simulink model "MIL4L3_SW6_V1_20220211"  (R2018b)
settings: Solver=FixedStepAuto  StartTime=0.0  StopTime=inf  FixedStep=0.001  RelTol=1e-3
PreLoadFcn:
  | A0_MILtest;
undefined symbols (not defined in the file or in its folder): Clb_ICADirect_LaneDisp_StateFive, Clb_ICADirect_LaneDisp_StateFour, Clb_ICADirect_LaneDisp_StateOne, Clb_ICADirect_LaneDisp_StateThree, Clb_ICADirect_LaneDisp_StateTwo, Clb_ICADirect_LaneDisp_StateZero, Clb_ICADirect_LaneDispSW, Clb_ICADirect_TrnLghtsCom_Switch, Clb_ICADirect_TrnLghtsCom_Value, Clb_ICADirect_TrnLghtsCrtl_Inhb, IMAP_Clb_ACU_Driver_Belt, IMAP_Clb_ACU_Driver_Belt_Over, IMAP_Clb_ACU_Passenger_Belt, IMAP_Clb_ACU_Passenger_Belt_Over, IMAP_Clb_ACU_RearLeft_Belt, IMAP_Clb_ACU_RearLeft_Belt_Over, IMAP_Clb_ACU_RearMiddle_Belt, IMAP_Clb_ACU_RearMiddle_Belt_Over, IMAP_Clb_ACU_RearRight_Belt, IMAP_Clb_ACU_RearRight_Belt_Over, IMAP_Clb_AEB_Switch, IMAP_Clb_AEB_Switch_Over, IMAP_Clb_ALC_TLC_Mode, IMAP_Clb_ALC_TLC_Mode_Over, IMAP_Clb_BCM_Battery_Voltage, IMAP_Clb_BCM_Battery_Voltage_Over, IMAP_Clb_BCM_BrakeLamp_State, IMAP_Clb_BCM_BrakeLamp_State_Over, IMAP_Clb_BCM_CHMSL_Status, IMAP_Clb_BCM_CHMSL_Status_Over, IMAP_Clb_BCM_Door_Lock_State, IMAP_Clb_BCM_Door_Lock_State_Over, IMAP_Clb_BCM_FrontWiper_State, IMAP_Clb_BCM_FrontWiper_State_Over, IMAP_Clb_BCM_FrontWiper_Switch, IMAP_Clb_BCM_FrontWiper_Switch_Over, IMAP_Clb_BCM_HazardLamp, IMAP_Clb_BCM_HazardLamp_Over, IMAP_Clb_BCM_HazardLamp_Switch, IMAP_Clb_BCM_HazardLamp_Switch_Over, IMAP_Clb_BCM_HighBeam_State, IMAP_Clb_BCM_HighBeam_State_Over, IMAP_Clb_BCM_Ignition_State, IMAP_Clb_BCM_Ignition_State_Over, IMAP_Clb_BCM_IHBC_Enabled, IMAP_Clb_BCM_IHBC_Enabled_Over, IMAP_Clb_BCM_Left_Light, IMAP_Clb_BCM_Left_Light_Over, IMAP_Clb_BCM_LeftTurn_Switch, IMAP_Clb_BCM_LeftTurn_Switch_Over, IMAP_Clb_BCM_LF_Door_State, IMAP_Clb_BCM_LF_Door_State_Over, IMAP_Clb_BCM_LowBeam_State, IMAP_Clb_BCM_LowBeam_State_Over, IMAP_Clb_BCM_LR_Door_State, IMAP_Clb_BCM_LR_Door_State_Over, IMAP_Clb_BCM_RF_Door_State, IMAP_Clb_BCM_RF_Door_State_Over, IMAP_Clb_BCM_Right_Light, IMAP_Clb_BCM_Right_Light_Over ... (+547)
libraries: CarMaker4SL x2153, simulink x292, dspstat3 x3, canmsglib x2, simulink_extras x1
(part 5 of 52)

== system MIL4L3_SW6_V1_20220211/CarMaker/VehicleControl/SwitchForRealECU_Steering_Angle ==
  In1 : Inport
  Inport : Inport  Port=2
  Compare To Constant1 : simulink/Logic and Bit Operations/Compare To Constant  relop===  const=2  OutDataTypeStr=boolean
  Compare To Constant2 : simulink/Logic and Bit Operations/Compare To Constant  relop===  const=4  OutDataTypeStr=boolean
  Define CM Dict3 : CarMaker4SL/Define CM Dict  xname=User.IO.In.SteeringAngle_Gain  xmono=off  xtype=Double4  xdvaplace=IO_In  xnstates=0  xfirststate=0  xinitial=1
  Define CM Dict4 : CarMaker4SL/Define CM Dict  xname=User.IO.In.SteeringAngle_SW  xmono=off  xtype=Double4  xdvaplace=IO_In  xnstates=0  xfirststate=0  xinitial=0
  Define CM Dict5 : CarMaker4SL/Define CM Dict  xname=User.IO.In.SteeringAngle_SW_Value  xmono=off  xtype=Double4  xdvaplace=IO_In  xnstates=0  xfirststate=0  xinitial=0
  Gain1 : Gain  Gain=pi/180
  Logical Operator : Logic  Operator=OR  AllPortsSameDT=off  OutDataTypeStr=boolean
  Product1 : Product
  Read CM Dict1 : CarMaker4SL/Read CM Dict  xname=User.IO.In.SteeringAngle_SW  xsync=off
  Read CM Dict2 : CarMaker4SL/Read CM Dict  xname=User.IO.In.SteeringAngle_Gain  xsync=off
  Read CM Dict3 : CarMaker4SL/Read CM Dict  xname=User.IO.In.SteeringAngle_SW_Value  xsync=off
  Read CM Dict4 : CarMaker4SL/Read CM Dict  xname=User.IO.In.ADAS_ICAStatusIcon  xsync=off
  Read CM Dict6 : CarMaker4SL/Read CM Dict  xname=User.IO.In.ADAS_LKAState  xsync=off
  Subsystem1 : Subsystem
  Switch1 : Switch  Criteria=u2 > Threshold  Threshold=0.5
  Switch2 : Switch  Criteria=u2 > Threshold  Threshold=0.5
  Out1 : Outport
  wires:
  In1/1 -> Switch1/3
  Read CM Dict4/1 -> Compare To Constant1/1
  Inport/1 -> Gain1/1
  Read CM Dict2/1 -> Product1/2
  Product1/1 -> Switch1/1
  Switch2/1 -> Out1/1
  Switch1/1 -> Switch2/3
  Read CM Dict1/1 -> Switch2/2
  Read CM Dict3/1 -> Switch2/1
  Gain1/1 -> Product1/1, Subsystem1/1(In1)
  Read CM Dict6/1 -> Compare To Constant2/1
  Compare To Constant1/1 -> Logical Operator/1
  Logical Operator/1 -> Switch1/2
  Compare To Constant2/1 -> Logical Operator/2

== system MIL4L3_SW6_V1_20220211/CarMaker/VehicleControl/SwitchForRealECU_Steering_Angle1 ==
  Torque : Inport
  User.IO.In.ADAS_ESATorqueReq : Inport  Port=2
  Compare To Constant1 : simulink/Logic and Bit Operations/Compare To Constant  relop===  const=4  OutDataTypeStr=boolean
  Read CM Dict4 : CarMaker4SL/Read CM Dict  xname=User.IO.In.ADAS_ESAState  xsync=off
  Switch1 : Switch  Criteria=u2 > Threshold  Threshold=0.5
  Out1 : Outport
  wires:
  User.IO.In.ADAS_ESATorqueReq/1 -> Switch1/1
  Compare To Constant1/1 -> Switch1/2
  Read CM Dict4/1 -> Compare To Constant1/1
  Switch1/1 -> Out1/1
  Torque/1 -> Switch1/3

== system MIL4L3_SW6_V1_20220211/CarMaker/VehicleControl/Traffic Attribution Define1 ==
  T00 : Subsystem
  T01 : Subsystem
  T02 : Subsystem
  T03 : Subsystem
  T04 : Subsystem
  T05 : Subsystem
  T06 : Subsystem
  T07 : Subsystem
  T08 : Subsystem
  T09 : Subsystem
  T10 : Subsystem
  T11 : Subsystem
  T12 : Subsystem
  T13 : Subsystem
  T14 : Subsystem
  T15 : Subsystem
  T16 : Subsystem
  T17 : Subsystem
  T18 : Subsystem
  T19 : Subsystem
  T20 : Subsystem
  T21 : Subsystem
  T22 : Subsystem
  T23 : Subsystem

== system MIL4L3_SW6_V1_20220211/CarMaker/VehicleControl/User.IO.In ==
  note: LKA
  note: JA
  note: FDMM
  note: AEB
  note: ESA
  note: EWWW
  note: ELK
  note: ACC
  Define CM Dict : CarMaker4SL/Define CM Dict  xname=User.IO.In.ACCSve_d_ACC_State  xmono=off  xtype=UInt  xdvaplace=None  xnstates=0  xfirststate=0  xinitial=0
  Define CM Dict1 : CarMaker4SL/Define CM Dict  xname=User.IO.In.ACCSve_g_ACC_DecReq  xmono=off  xtype=UInt  xdvaplace=None  xnstates=0  xfirststate=0  xinitial=0
  Define CM Dict10 : CarMaker4SL/Define CM Dict  xname=User.IO.In.ACCSva_d_ACCS2ICAB  xmono=off  xtype=UInt  xdvaplace=None  xnstates=0  xfirststate=0  xinitial=0
  Define CM Dict100 : CarMaker4SL/Define CM Dict  xname=User.IO.In.LKASve_y_LDW_Status_Display  xmono=off  xtype=UInt  xdvaplace=None  xnstates=0  xfirststate=0  xinitial=0
  Define CM Dict101 : CarMaker4SL/Define CM Dict  xname=User.IO.In.LKASve_y_LKA_Status_Display  xmono=off  xtype=UInt  xdvaplace=None  xnstates=0  xfirststate=0  xinitial=0
  Define CM Dict102 : CarMaker4SL/Define CM Dict  xname=User.IO.In.LKASve_y_Hands_Off_Warning  xmono=off  xtype=UInt  xdvaplace=None  xnstates=0  xfirststate=0  xinitial=0
  Define CM Dict103 : CarMaker4SL/Define CM Dict  xname=User.IO.In.LKASve_y_LKA_Action_Indication  xmono=off  xtype=UInt  xdvaplace=None  xnstates=0  xfirststate=0  xinitial=0
  Define CM Dict104 : CarMaker4SL/Define CM Dict  xname=User.IO.In.LKASve_g_LKA_SWA_Control  xmono=off  xtype=UInt  xdvaplace=None  xnstates=0  xfirststate=0  xinitial=0
  Define CM Dict105 : CarMaker4SL/Define CM Dict  xname=User.IO.In.LKASve_y_HMI_Popup_Status  xmono=off  xtype=UInt  xdvaplace=None  xnstates=0  xfirststate=0  xinitial=0
  Define CM Dict106 : CarMaker4SL/Define CM Dict  xname=User.IO.In.LKASve_y_EPS_State_Control  xmono=off  xtype=UInt  xdvaplace=None  xnstates=0  xfirststate=0  xinitial=0
  Define CM Dict107 : CarMaker4SL/Define CM Dict  xname=User.IO.In.LKASve_g_EPS_Factor_Control  xmono=off  xtype=UInt  xdvaplace=None  xnstates=0  xfirststate=0  xinitial=0
  Define CM Dict11 : CarMaker4SL/Define CM Dict  xname=User.IO.In.ELKSve_y_state_ELK function  xmono=off  xtype=UInt  xdvaplace=None  xnstates=0  xfirststate=0  xinitial=0
  Define CM Dict12 : CarMaker4SL/Define CM Dict  xname=User.IO.In.ACCSve_g_SignalTStamp  xmono=off  xtype=UInt  xdvaplace=None  xnstates=0  xfirststate=0  xinitial=0
  Define CM Dict13 : CarMaker4SL/Define CM Dict  xname=User.IO.In.ELKSve_y_HMI_Popup_Status  xmono=off  xtype=UInt  xdvaplace=None  xnstates=0  xfirststate=0  xinitial=0
  Define CM Dict14 : CarMaker4SL/Define CM Dict  xname=User.IO.In.ESASve_y_EPS_State  xmono=off  xtype=UInt  xdvaplace=None  xnstates=0  xfirststate=0  xinitial=0
  Define CM Dict15 : CarMaker4SL/Define CM Dict  xname=User.IO.In.ESASve_g_SignalTStamp  xmono=off  xtype=UInt  xdvaplace=None  xnstates=0  xfirststate=0  xinitial=0
  Define CM Dict16 : CarMaker4SL/Define CM Dict  xname=User.IO.In.ELKSve_b_Hands_Off_Warning  xmono=off  xtype=UInt  xdvaplace=None  xnstates=0  xfirststate=0  xinitial=0
  Define CM Dict17 : CarMaker4SL/Define CM Dict  xname=User.IO.In.ELKSve_y_ELK_Action_Indication  xmono=off  xtype=UInt  xdvaplace=None  xnstates=0  xfirststate=0  xinitial=0
  Define CM Dict18 : CarMaker4SL/Define CM Dict  xname=User.IO.In.ELKSve_y_EPS_State_Control  xmono=off  xtype=UInt  xdvaplace=None  xnstates=0  xfirststate=0  xinitial=0
  Define CM Dict19 : CarMaker4SL/Define CM Dict  xname=User.IO.In.ELKSve_g_ELK_SWA_Control  xmono=off  xtype=UInt  xdvaplace=None  xnstates=0  xfirststate=0  xinitial=0
  Define CM Dict2 : CarMaker4SL/Define CM Dict  xname=User.IO.In.ACCSve_g_ACC_TqReq  xmono=off  xtype=UInt  xdvaplace=None  xnstates=0  xfirststate=0  xinitial=0
  Define CM Dict20 : CarMaker4SL/Define CM Dict  xname=User.IO.In.ELKSve_g_SignalTStamp  xmono=off  xtype=UInt  xdvaplace=None  xnstates=0  xfirststate=0  xinitial=0
  Define CM Dict21 : CarMaker4SL/Define CM Dict  xname=User.IO.In.ELKSve_g_EPS_Factor_Control  xmono=off  xtype=UInt  xdvaplace=None  xnstates=0  xfirststate=0  xinitial=0
  Define CM Dict22 : CarMaker4SL/Define CM Dict  xname=User.IO.In.ELKSve_b_EPS_ELK_Control  xmono=off  xtype=UInt  xdvaplace=None  xnstates=0  xfirststate=0  xinitial=0
  Define CM Dict23 : CarMaker4SL/Define CM Dict  xname=User.IO.In.AEBSve_d_Prefill_request  xmono=off  xtype=UInt  xdvaplace=None  xnstates=0  xfirststate=0  xinitial=0
  Define CM Dict24 : CarMaker4SL/Define CM Dict  xname=User.IO.In.AEBSve_d_MDDdecRequest  xmono=off  xtype=UInt  xdvaplace=None  xnstates=0  xfirststate=0  xinitial=0
  Define CM Dict25 : CarMaker4SL/Define CM Dict  xname=User.IO.In.ESASve_g_ESA_SWA_CMD  xmono=off  xtype=UInt  xdvaplace=None  xnstates=0  xfirststate=0  xinitial=0
  Define CM Dict26 : CarMaker4SL/Define CM Dict  xname=User.IO.In.ESASve_g_EPS_Factor_Control  xmono=off  xtype=UInt  xdvaplace=None  xnstates=0  xfirststate=0  xinitial=0
  Define CM Dict27 : CarMaker4SL/Define CM Dict  xname=User.IO.In.AEBSve_d_AEBFaultStatus  xmono=off  xtype=UInt  xdvaplace=None  xnstates=0  xfirststate=0  xinitial=0
  Define CM Dict28 : CarMaker4SL/Define CM Dict  xname=User.IO.In.AEBSve_d_AEBAlertReq  xmono=off  xtype=UInt  xdvaplace=None  xnstates=0  xfirststate=0  xinitial=0
  Define CM Dict29 : CarMaker4SL/Define CM Dict  xname=User.IO.In.AEBSve_d_functionFARCState  xmono=off  xtype=UInt  xdvaplace=None  xnstates=0  xfirststate=0  xinitial=0
  Define CM Dict3 : CarMaker4SL/Define CM Dict  xname=User.IO.In.ACCSve_d_ACC_TqFlag  xmono=off  xtype=UInt  xdvaplace=None  xnstates=0  xfirststate=0  xinitial=0
  Define CM Dict30 : CarMaker4SL/Define CM Dict  xname=User.IO.In.AEBSve_g_DecSetpoint  xmono=off  xtype=UInt  xdvaplace=None  xnstates=0  xfirststate=0  xinitial=0
  Define CM Dict31 : CarMaker4SL/Define CM Dict  xname=User.IO.In.AEBSve_d_MDDdecType  xmono=off  xtype=UInt  xdvaplace=None  xnstates=0  xfirststate=0  xinitial=0
  Define CM Dict32 : CarMaker4SL/Define CM Dict  xname=User.IO.In.AEBSve_d_HapticAlarm  xmono=off  xtype=UInt  xdvaplace=None  xnstates=0  xfirststate=0  xinitial=0
  Define CM Dict33 : CarMaker4SL/Define CM Dict  xname=User.IO.In.AEBSve_d_FCWStatus  xmono=off  xtype=UInt  xdvaplace=None  xnstates=0  xfirststate=0  xinitial=0
  Define CM Dict34 : CarMaker4SL/Define CM Dict  xname=User.IO.In.AEBSve_d_Braking_progress  xmono=off  xtype=UInt  xdvaplace=None  xnstates=0  xfirststate=0  xinitial=0
  Define CM Dict35 : CarMaker4SL/Define CM Dict  xname=User.IO.In.AEBSve_d_AEBStatus  xmono=off  xtype=UInt  xdvaplace=None  xnstates=0  xfirststate=0  xinitial=0
  Define CM Dict36 : CarMaker4SL/Define CM Dict  xname=User.IO.In.AEBSve_d_AEBSwitchStatus  xmono=off  xtype=UInt  xdvaplace=None  xnstates=0  xfirststate=0  xinitial=0
  Define CM Dict37 : CarMaker4SL/Define CM Dict  xname=User.IO.In.AEBSve_g_SignalTStamp  xmono=off  xtype=UInt  xdvaplace=None  xnstates=0  xfirststate=0  xinitial=0
  Define CM Dict38 : CarMaker4SL/Define CM Dict  xname=User.IO.In.AEBSve_d_AEBTips  xmono=off  xtype=UInt  xdvaplace=None  xnstates=0  xfirststate=0  xinitial=0
  Define CM Dict39 : CarMaker4SL/Define CM Dict  xname=User.IO.In.JABSve_d_AlertSign  xmono=off  xtype=UInt  xdvaplace=None  xnstates=0  xfirststate=0  xinitial=0
  Define CM Dict4 : CarMaker4SL/Define CM Dict  xname=User.IO.In.ACCSve_d_ACC_DecFlag  xmono=off  xtype=UInt  xdvaplace=None  xnstates=0  xfirststate=0  xinitial=0
  Define CM Dict40 : CarMaker4SL/Define CM Dict  xname=User.IO.In.EWWWve_y_LCW_M_SystemWorkingSt  xmono=off  xtype=UInt  xdvaplace=None  xnstates=0  xfirststate=0  xinitial=0
  Define CM Dict41 : CarMaker4SL/Define CM Dict  xname=User.IO.In.EWWWve_y_BSD_M_ErrorSt  xmono=off  xtype=UInt  xdvaplace=None  xnstates=0  xfirststate=0  xinitial=0
  Define CM Dict42 : CarMaker4SL/Define CM Dict  xname=User.IO.In.JABSve_d_SwitchStatus  xmono=off  xtype=UInt  xdvaplace=None  xnstates=0  xfirststate=0  xinitial=0
  Define CM Dict43 : CarMaker4SL/Define CM Dict  xname=User.IO.In.JABSve_d_HapticAlarm  xmono=off  xtype=UInt  xdvaplace=None  xnstates=0  xfirststate=0  xinitial=0
  Define CM Dict44 : CarMaker4SL/Define CM Dict  xname=User.IO.In.JABSve_d_FltStatus  xmono=off  xtype=UInt  xdvaplace=None  xnstates=0  xfirststate=0  xinitial=0
  Define CM Dict45 : CarMaker4SL/Define CM Dict  xname=User.IO.In.JABSve_d_AlertReq  xmono=off  xtype=UInt  xdvaplace=None  xnstates=0  xfirststate=0  xinitial=0
  Define CM Dict46 : CarMaker4SL/Define CM Dict  xname=User.IO.In.JABSve_d_Tips  xmono=off  xtype=UInt  xdvaplace=None  xnstates=0  xfirststate=0  xinitial=0
  Define CM Dict47 : CarMaker4SL/Define CM Dict  xname=User.IO.In.EWWWve_y_BSD_S_ErrorSt  xmono=off  xtype=UInt  xdvaplace=None  xnstates=0  xfirststate=0  xinitial=0
  Define CM Dict48 : CarMaker4SL/Define CM Dict  xname=User.IO.In.EWWWve_y_BSD_S_LCAWarning  xmono=off  xtype=UInt  xdvaplace=None  xnstates=0  xfirststate=0  xinitial=0
  Define CM Dict49 : CarMaker4SL/Define CM Dict  xname=User.IO.In.EWWWve_y_RCTA_M_SystemWorkingSt  xmono=off  xtype=UInt  xdvaplace=None  xnstates=0  xfirststate=0  xinitial=0
  Define CM Dict5 : CarMaker4SL/Define CM Dict  xname=User.IO.In.ACCSve_d_CIPV_ID  xmono=off  xtype=UInt  xdvaplace=None  xnstates=0  xfirststate=0  xinitial=0
  Define CM Dict50 : CarMaker4SL/Define CM Dict  xname=User.IO.In.EWWWve_y_DOW_M_SystemWorkingSt  xmono=off  xtype=UInt  xdvaplace=None  xnstates=0  xfirststate=0  xinitial=0
  Define CM Dict51 : CarMaker4SL/Define CM Dict  xname=User.IO.In.EWWWve_y_BSD_M_LCAWarning  xmono=off  xtype=UInt  xdvaplace=None  xnstates=0  xfirststate=0  xinitial=0
  Define CM Dict52 : CarMaker4SL/Define CM Dict  xname=User.IO.In.EWWWve_y_BSD_M_DoorOpenWarning  xmono=off  xtype=UInt  xdvaplace=None  xnstates=0  xfirststate=0  xinitial=0
  Define CM Dict53 : CarMaker4SL/Define CM Dict  xname=User.IO.In.EWWWve_y_RCTA_S_SystemWorkingSt  xmono=off  xtype=UInt  xdvaplace=None  xnstates=0  xfirststate=0  xinitial=0
  Define CM Dict54 : CarMaker4SL/Define CM Dict  xname=User.IO.In.EWWWve_y_BSD_M_RCTAWarning  xmono=off  xtype=UInt  xdvaplace=None  xnstates=0  xfirststate=0  xinitial=0
  Define CM Dict55 : CarMaker4SL/Define CM Dict  xname=User.IO.In.EWWWve_y_LCW_S_SystemWorkingSt  xmono=off  xtype=UInt  xdvaplace=None  xnstates=0  xfirststate=0  xinitial=0
  Define CM Dict56 : CarMaker4SL/Define CM Dict  xname=User.IO.In.EWWWve_y_DOW_S_SystemWorkingSt  xmono=off  xtype=UInt  xdvaplace=None  xnstates=0  xfirststate=0  xinitial=0
  Define CM Dict57 : CarMaker4SL/Define CM Dict  xname=User.IO.In.EWWWve_y_BSD_S_RCTAWarning  xmono=off  xtype=UInt  xdvaplace=None  xnstates=0  xfirststate=0  xinitial=0
  Define CM Dict58 : CarMaker4SL/Define CM Dict  xname=User.IO.In.EWWWve_y_BSD_S_DoorOpenWarning  xmono=off  xtype=UInt  xdvaplace=None  xnstates=0  xfirststate=0  xinitial=0
  Define CM Dict59 : CarMaker4SL/Define CM Dict  xname=User.IO.In.EWWWve_y_FCTA_L_SystemWorkingSt  xmono=off  xtype=UInt  xdvaplace=None  xnstates=0  xfirststate=0  xinitial=0
  Define CM Dict6 : CarMaker4SL/Define CM Dict  xname=User.IO.In.ACCSve_d_VelocitySet  xmono=off  xtype=UInt  xdvaplace=None  xnstates=0  xfirststate=0  xinitial=0
  Define CM Dict60 : CarMaker4SL/Define CM Dict  xname=User.IO.In.EWWWve_y_SRR_LF_ErrorSt  xmono=off  xtype=UInt  xdvaplace=None  xnstates=0  xfirststate=0  xinitial=0
  Define CM Dict61 : CarMaker4SL/Define CM Dict  xname=User.IO.In.EWWWve_y_SRR_RF_ErrorSt  xmono=off  xtype=UInt  xdvaplace=None  xnstates=0  xfirststate=0  xinitial=0
  Define CM Dict62 : CarMaker4SL/Define CM Dict  xname=User.IO.In.EWWWve_y_SRR_LF_FCTAWarning  xmono=off  xtype=UInt  xdvaplace=None  xnstates=0  xfirststate=0  xinitial=0
  Define CM Dict63 : CarMaker4SL/Define CM Dict  xname=User.IO.In.EWWWve_y_FCTA_R_SystemWorkingSt  xmono=off  xtype=UInt  xdvaplace=None  xnstates=0  xfirststate=0  xinitial=0
  Define CM Dict64 : CarMaker4SL/Define CM Dict  xname=User.IO.In.EWWWve_y_SRR_RF_FCTAWarning  xmono=off  xtype=UInt  xdvaplace=None  xnstates=0  xfirststate=0  xinitial=0
  Define CM Dict65 : CarMaker4SL/Define CM Dict  xname=User.IO.In.EWWWve_y_FCTA_InitResult  xmono=off  xtype=UInt  xdvaplace=None  xnstates=0  xfirststate=0  xinitial=0
  Define CM Dict66 : CarMaker4SL/Define CM Dict  xname=User.IO.In.FDMMve_d_JaFcnConf  xmono=off  xtype=UInt  xdvaplace=None  xnstates=0  xfirststate=0  xinitial=0
  Define CM Dict67 : CarMaker4SL/Define CM Dict  xname=User.IO.In.EWWWve_y_BSD_InitResult  xmono=off  xtype=UInt  xdvaplace=None  xnstates=0  xfirststate=0  xinitial=0
  Define CM Dict68 : CarMaker4SL/Define CM Dict  xname=User.IO.In.EWWWve_y_SRR_SystemState  xmono=off  xtype=UInt  xdvaplace=None  xnstates=0  xfirststate=0  xinitial=0
  Define CM Dict69 : CarMaker4SL/Define CM Dict  xname=User.IO.In.FDMMve_d_ElkFcnConf  xmono=off  xtype=UInt  xdvaplace=None  xnstates=0  xfirststate=0  xinitial=0
  Define CM Dict7 : CarMaker4SL/Define CM Dict  xname=User.IO.In.ACCSve_d_ACCActive_Signal  xmono=off  xtype=UInt  xdvaplace=None  xnstates=0  xfirststate=0  xinitial=0
  Define CM Dict70 : CarMaker4SL/Define CM Dict  xname=User.IO.In.FDMMve_g_Adas2Fapa  xmono=off  xtype=UInt  xdvaplace=None  xnstates=0  xfirststate=0  xinitial=0
  Define CM Dict71 : CarMaker4SL/Define CM Dict  xname=User.IO.In.FDMMve_g_SignalTStamp  xmono=off  xtype=UInt  xdvaplace=None  xnstates=0  xfirststate=0  xinitial=0
  Define CM Dict72 : CarMaker4SL/Define CM Dict  xname=User.IO.In.FDMMve_d_AebFcnConf  xmono=off  xtype=UInt  xdvaplace=None  xnstates=0  xfirststate=0  xinitial=0
  Define CM Dict73 : CarMaker4SL/Define CM Dict  xname=User.IO.In.FDMMve_d_EsaFcnConf  xmono=off  xtype=UInt  xdvaplace=None  xnstates=0  xfirststate=0  xinitial=0
  Define CM Dict74 : CarMaker4SL/Define CM Dict  xname=User.IO.In.FDMMve_d_LkaFcnConf  xmono=off  xtype=UInt  xdvaplace=None  xnstates=0  xfirststate=0  xinitial=0
  Define CM Dict75 : CarMaker4SL/Define CM Dict  xname=User.IO.In.FDMMve_d_IcaFcnConf  xmono=off  xtype=UInt  xdvaplace=None  xnstates=0  xfirststate=0  xinitial=0
  Define CM Dict76 : CarMaker4SL/Define CM Dict  xname=User.IO.In.FDMMve_d_AlcFcnConf  xmono=off  xtype=UInt  xdvaplace=None  xnstates=0  xfirststate=0  xinitial=0
  Define CM Dict77 : CarMaker4SL/Define CM Dict  xname=User.IO.In.FDMMve_d_AccFcnConf  xmono=off  xtype=UInt  xdvaplace=None  xnstates=0  xfirststate=0  xinitial=0
  Define CM Dict78 : CarMaker4SL/Define CM Dict  xname=User.IO.In.FDMMve_d_LfFcnConf  xmono=off  xtype=UInt  xdvaplace=None  xnstates=0  xfirststate=0  xinitial=0
  Define CM Dict79 : CarMaker4SL/Define CM Dict  xname=User.IO.In.FDMMve_d_EwFcnConf  xmono=off  xtype=UInt  xdvaplace=None  xnstates=0  xfirststate=0  xinitial=0
  Define CM Dict8 : CarMaker4SL/Define CM Dict  xname=User.IO.In.ACCSve_d_ACC_go_request  xmono=off  xtype=UInt  xdvaplace=None  xnstates=0  xfirststate=0  xinitial=0
  Define CM Dict80 : CarMaker4SL/Define CM Dict  xname=User.IO.In.JABSve_d_Switching  xmono=off  xtype=UInt  xdvaplace=None  xnstates=0  xfirststate=0  xinitial=0
  Define CM Dict81 : CarMaker4SL/Define CM Dict  xname=User.IO.In.JABSve_y_Prefill_request  xmono=off  xtype=UInt  xdvaplace=None  xnstates=0  xfirststate=0  xinitial=0
  Define CM Dict82 : CarMaker4SL/Define CM Dict  xname=User.IO.In.JABSve_d_DbAlertSign  xmono=off  xtype=UInt  xdvaplace=None  xnstates=0  xfirststate=0  xinitial=0
  Define CM Dict83 : CarMaker4SL/Define CM Dict  xname=User.IO.In.JABSve_d_DbSwitchStatus  xmono=off  xtype=UInt  xdvaplace=None  xnstates=0  xfirststate=0  xinitial=0
  Define CM Dict84 : CarMaker4SL/Define CM Dict  xname=User.IO.In.JABSve_a_DecelReq  xmono=off  xtype=UInt  xdvaplace=None  xnstates=0  xfirststate=0  xinitial=0
  Define CM Dict85 : CarMaker4SL/Define CM Dict  xname=User.IO.In.JABSve_g_SignalTStamp  xmono=off  xtype=UInt  xdvaplace=None  xnstates=0  xfirststate=0  xinitial=0
  Define CM Dict86 : CarMaker4SL/Define CM Dict  xname=User.IO.In.JABSve_y_functionFARCState  xmono=off  xtype=UInt  xdvaplace=None  xnstates=0  xfirststate=0  xinitial=0
  Define CM Dict87 : CarMaker4SL/Define CM Dict  xname=User.IO.In.JABSve_a_DecSetpoint  xmono=off  xtype=UInt  xdvaplace=None  xnstates=0  xfirststate=0  xinitial=0
  Define CM Dict88 : CarMaker4SL/Define CM Dict  xname=User.IO.In.JABSve_y_HapticAlarm  xmono=off  xtype=UInt  xdvaplace=None  xnstates=0  xfirststate=0  xinitial=0
  Define CM Dict89 : CarMaker4SL/Define CM Dict  xname=User.IO.In.JABSve_y_MDDdecRequest  xmono=off  xtype=UInt  xdvaplace=None  xnstates=0  xfirststate=0  xinitial=0
  Define CM Dict9 : CarMaker4SL/Define CM Dict  xname=User.IO.In.ACCSve_d_HeadWaySet  xmono=off  xtype=UInt  xdvaplace=None  xnstates=0  xfirststate=0  xinitial=0
  Define CM Dict90 : CarMaker4SL/Define CM Dict  xname=User.IO.In.JABSve_y_MDDdecType  xmono=off  xtype=UInt  xdvaplace=None  xnstates=0  xfirststate=0  xinitial=0
  Define CM Dict91 : CarMaker4SL/Define CM Dict  xname=User.IO.In.JABSve_g_DbSignalTStamp  xmono=off  xtype=UInt  xdvaplace=None  xnstates=0  xfirststate=0  xinitial=0
  Define CM Dict92 : CarMaker4SL/Define CM Dict  xname=User.IO.In.JABSve_d_DbTAlertReq  xmono=off  xtype=UInt  xdvaplace=None  xnstates=0  xfirststate=0  xinitial=0
  Define CM Dict93 : CarMaker4SL/Define CM Dict  xname=User.IO.In.JABSve_d_DbFltStatus  xmono=off  xtype=UInt  xdvaplace=None  xnstates=0  xfirststate=0  xinitial=0
  Define CM Dict94 : CarMaker4SL/Define CM Dict  xname=User.IO.In.JABSve_d_DbHapticAlarm  xmono=off  xtype=UInt  xdvaplace=None  xnstates=0  xfirststate=0  xinitial=0
  Define CM Dict95 : CarMaker4SL/Define CM Dict  xname=User.IO.In.JABSve_d_DbTips  xmono=off  xtype=UInt  xdvaplace=None  xnstates=0  xfirststate=0  xinitial=0
  Define CM Dict96 : CarMaker4SL/Define CM Dict  xname=User.IO.In.LKASve_y_Vehicle_Lane_Display  xmono=off  xtype=UInt  xdvaplace=None  xnstates=0  xfirststate=0  xinitial=0
  Define CM Dict97 : CarMaker4SL/Define CM Dict  xname=User.IO.In.LKASve_y_LDW_Flag  xmono=off  xtype=UInt  xdvaplace=None  xnstates=0  xfirststate=0  xinitial=0
  Define CM Dict98 : CarMaker4SL/Define CM Dict  xname=User.IO.In.LKASve_y_EPS_LKA_Control  xmono=off  xtype=UInt  xdvaplace=None  xnstates=0  xfirststate=0  xinitial=0

== system MIL4L3_SW6_V1_20220211/CarMaker/VehicleControl/User.IO.Out ==
  ActuatorStatus2Ctrl : Subsystem
  Define CM Dict : CarMaker4SL/Define CM Dict  xname=User.IO.Out.Mp5_LKA_main_SW  xmono=off  xtype=UInt  xdvaplace=None  xnstates=0  xfirststate=0  xinitial=0
  Define CM Dict1 : CarMaker4SL/Define CM Dict  xname=User.IO.Out.Mp5_LKA_Mode  xmono=off  xtype=UInt  xdvaplace=None  xnstates=0  xfirststate=0  xinitial=0
  Define CM Dict10 : CarMaker4SL/Define CM Dict  xname=User.IO.Out.MP5_ALCTLC_Mode  xmono=off  xtype=UInt  xdvaplace=None  xnstates=0  xfirststate=0  xinitial=0
  Define CM Dict11 : CarMaker4SL/Define CM Dict  xname=User.IO.Out.Mp5_ESA_Cfg  xmono=off  xtype=UInt  xdvaplace=None  xnstates=0  xfirststate=0  xinitial=0
  Define CM Dict12 : CarMaker4SL/Define CM Dict  xname=User.IO.Out.Mp5_ELK_Cfg  xmono=off  xtype=UInt  xdvaplace=None  xnstates=0  xfirststate=0  xinitial=0
  Define CM Dict13 : CarMaker4SL/Define CM Dict  xname=User.IO.Out.AutoParkingCmd  xmono=off  xtype=UInt  xdvaplace=None  xnstates=0  xfirststate=0  xinitial=0
  Define CM Dict14 : CarMaker4SL/Define CM Dict  xname=User.IO.Out.LFConf  xmono=off  xtype=UInt  xdvaplace=None  xnstates=0  xfirststate=0  xinitial=0
  Define CM Dict15 : CarMaker4SL/Define CM Dict  xname=User.IO.Out.ICAConf  xmono=off  xtype=UInt  xdvaplace=None  xnstates=0  xfirststate=0  xinitial=0
  Define CM Dict16 : CarMaker4SL/Define CM Dict  xname=User.IO.Out.PEPS_RKECommand  xmono=off  xtype=UInt  xdvaplace=None  xnstates=0  xfirststate=0  xinitial=0
  Define CM Dict17 : CarMaker4SL/Define CM Dict  xname=User.IO.Out.MP5_BSD_LCW_ACT  xmono=off  xtype=UInt  xdvaplace=None  xnstates=0  xfirststate=0  xinitial=0
  Define CM Dict18 : CarMaker4SL/Define CM Dict  xname=User.IO.Out.MP5_FCTA_ACT  xmono=off  xtype=UInt  xdvaplace=None  xnstates=0  xfirststate=0  xinitial=0
  Define CM Dict19 : CarMaker4SL/Define CM Dict  xname=User.IO.Out.MP5_RCTA_ACT  xmono=off  xtype=UInt  xdvaplace=None  xnstates=0  xfirststate=0  xinitial=0
  Define CM Dict2 : CarMaker4SL/Define CM Dict  Commented=on  xname=User.IO.Out.MP5_AEBSwitch  xmono=off  xtype=UInt  xdvaplace=None  xnstates=0  xfirststate=0  xinitial=0
  Define CM Dict20 : CarMaker4SL/Define CM Dict  xname=User.IO.Out.MP5_DOW_ACT  xmono=off  xtype=UInt  xdvaplace=None  xnstates=0  xfirststate=0  xinitial=0
  Define CM Dict21 : CarMaker4SL/Define CM Dict  xname=User.IO.Out.JaBrakConf  xmono=off  xtype=UInt  xdvaplace=None  xnstates=0  xfirststate=0  xinitial=0
  Define CM Dict22 : CarMaker4SL/Define CM Dict  xname=User.IO.Out.JaAlertConf  xmono=off  xtype=UInt  xdvaplace=None  xnstates=0  xfirststate=0  xinitial=0
  Define CM Dict23 : CarMaker4SL/Define CM Dict  xname=User.IO.Out.JaAlertSens  xmono=off  xtype=UInt  xdvaplace=None  xnstates=0  xfirststate=0  xinitial=0
  Define CM Dict24 : CarMaker4SL/Define CM Dict  xname=User.IO.Out.AlcSens  xmono=off  xtype=UInt  xdvaplace=None  xnstates=0  xfirststate=0  xinitial=0
  Define CM Dict25 : CarMaker4SL/Define CM Dict  xname=User.IO.Out.EPSErrSt  xmono=off  xtype=UInt  xdvaplace=None  xnstates=0  xfirststate=0  xinitial=0
  Define CM Dict26 : CarMaker4SL/Define CM Dict  xname=User.IO.Out.EPS_SteeringTrqS  xmono=off  xtype=UInt  xdvaplace=None  xnstates=0  xfirststate=0  xinitial=0.5
  Define CM Dict27 : CarMaker4SL/Define CM Dict  xname=User.IO.Out.ESC_ayv_valid  xmono=off  xtype=UInt  xdvaplace=None  xnstates=0  xfirststate=0  xinitial=0
  Define CM Dict28 : CarMaker4SL/Define CM Dict  xname=User.IO.Out.ESC_YawRate_valid  xmono=off  xtype=UInt  xdvaplace=None  xnstates=0  xfirststate=0  xinitial=0
  Define CM Dict29 : CarMaker4SL/Define CM Dict  xname=User.IO.Out.ESC_LonAcc_valid  xmono=off  xtype=UInt  xdvaplace=None  xnstates=0  xfirststate=0  xinitial=0
  Define CM Dict3 : CarMaker4SL/Define CM Dict  Commented=on  xname=User.IO.Out.MP5_FCWSwitch  xmono=off  xtype=UInt  xdvaplace=None  xnstates=0  xfirststate=0  xinitial=0
  Define CM Dict30 : CarMaker4SL/Define CM Dict  xname=User.IO.Out.BCM_Openingstates  xmono=off  xtype=UInt  xdvaplace=None  xnstates=0  xfirststate=0  xinitial=0
  Define CM Dict31 : CarMaker4SL/Define CM Dict  xname=User.IO.Out.BCM_TrunkSt  xmono=off  xtype=UInt  xdvaplace=None  xnstates=0  xfirststate=0  xinitial=0
  Define CM Dict32 : CarMaker4SL/Define CM Dict  xname=User.IO.Out.BCM_HazardLampSt  xmono=off  xtype=UInt  xdvaplace=None  xnstates=0  xfirststate=0  xinitial=0
  Define CM Dict33 : CarMaker4SL/Define CM Dict  xname=User.IO.Out.BCM_LetfligthSt  xmono=off  xtype=UInt  xdvaplace=None  xnstates=0  xfirststate=0  xinitial=0
  Define CM Dict34 : CarMaker4SL/Define CM Dict  xname=User.IO.Out.BCM_RightligthSt  xmono=off  xtype=UInt  xdvaplace=None  xnstates=0  xfirststate=0  xinitial=0
  Define CM Dict35 : CarMaker4SL/Define CM Dict  xname=User.IO.Out.ESC_BLRequest  xmono=off  xtype=UInt  xdvaplace=None  xnstates=0  xfirststate=0  xinitial=0
  Define CM Dict36 : CarMaker4SL/Define CM Dict  xname=User.IO.Out.BCM_LFDoorSt  xmono=off  xtype=UInt  xdvaplace=None  xnstates=0  xfirststate=0  xinitial=0
  Define CM Dict37 : CarMaker4SL/Define CM Dict  xname=User.IO.Out.BCM_RFDoorSt  xmono=off  xtype=UInt  xdvaplace=None  xnstates=0  xfirststate=0  xinitial=0
  Define CM Dict38 : CarMaker4SL/Define CM Dict  xname=User.IO.Out.BCM_RRDoorSt  xmono=off  xtype=UInt  xdvaplace=None  xnstates=0  xfirststate=0  xinitial=0
  Define CM Dict39 : CarMaker4SL/Define CM Dict  xname=User.IO.Out.BCM_LRDoorSt  xmono=off  xtype=UInt  xdvaplace=None  xnstates=0  xfirststate=0  xinitial=0
  Define CM Dict4 : CarMaker4SL/Define CM Dict  xname=User.IO.Out.MP5_FCW_Sensi  xmono=off  xtype=UInt  xdvaplace=None  xnstates=0  xfirststate=0  xinitial=0
  Define CM Dict40 : CarMaker4SL/Define CM Dict  xname=User.IO.Out.SCC_LeftSwSig  xmono=off  xtype=UInt  xdvaplace=None  xnstates=0  xfirststate=0  xinitial=0
  Define CM Dict41 : CarMaker4SL/Define CM Dict  xname=User.IO.Out.SCC_RightSwSig  xmono=off  xtype=UInt  xdvaplace=None  xnstates=0  xfirststate=0  xinitial=0
  Define CM Dict42 : CarMaker4SL/Define CM Dict  xname=User.IO.Out.GW_EMS_AccPedal  xmono=off  xtype=UInt  xdvaplace=None  xnstates=0  xfirststate=0  xinitial=0
  Define CM Dict43 : CarMaker4SL/Define CM Dict  xname=User.IO.Out.GW_EMS_AccPedFlt  xmono=off  xtype=Int  xdvaplace=None  xnstates=0  xfirststate=0  xinitial=0
  Define CM Dict44 : CarMaker4SL/Define CM Dict  xname=User.IO.Out.EPS_LKAState  xmono=off  xtype=UInt  xdvaplace=None  xnstates=0  xfirststate=0  xinitial=0
  Define CM Dict45 : CarMaker4SL/Define CM Dict  xname=User.IO.Out.BCM_DoorLockSt  xmono=off  xtype=UInt  xdvaplace=None  xnstates=0  xfirststate=0  xinitial=0
  Define CM Dict46 : CarMaker4SL/Define CM Dict  xname=User.IO.Out.EMS_Status_ACC  xmono=off  xtype=UInt  xdvaplace=None  xnstates=0  xfirststate=0  xinitial=0
  Define CM Dict47 : CarMaker4SL/Define CM Dict  xname=User.IO.Out.EMS_AccPedalR  xmono=off  xtype=UInt  xdvaplace=None  xnstates=0  xfirststate=0  xinitial=0
  Define CM Dict48 : CarMaker4SL/Define CM Dict  xname=User.IO.Out.BCM_IgnitionSt  xmono=off  xtype=UInt  xdvaplace=None  xnstates=0  xfirststate=0  xinitial=0
  Define CM Dict49 : CarMaker4SL/Define CM Dict  xname=User.IO.Out.ACU_DriverBelt  xmono=off  xtype=UInt  xdvaplace=None  xnstates=0  xfirststate=0  xinitial=0
  Define CM Dict5 : CarMaker4SL/Define CM Dict  xname=User.IO.Out.Mp5_ISA_Switch  xmono=off  xtype=UInt  xdvaplace=None  xnstates=0  xfirststate=0  xinitial=0
  Define CM Dict50 : CarMaker4SL/Define CM Dict  xname=User.IO.Out.SWS_fault_code  xmono=off  xtype=UInt  xdvaplace=None  xnstates=0  xfirststate=0  xinitial=0
  Define CM Dict51 : CarMaker4SL/Define CM Dict  xname=User.IO.Out.ESC_ESCOFF  xmono=off  xtype=UInt  xdvaplace=None  xnstates=0  xfirststate=0  xinitial=0
  Define CM Dict52 : CarMaker4SL/Define CM Dict  xname=User.IO.Out.GW_Speed_Lim_On  xmono=off  xtype=UInt  xdvaplace=None  xnstates=0  xfirststate=0  xinitial=0
  Define CM Dict53 : CarMaker4SL/Define CM Dict  xname=User.IO.Out.ESC_VehSpdValid  xmono=off  xtype=UInt  xdvaplace=None  xnstates=0  xfirststate=0  xinitial=0
  Define CM Dict54 : CarMaker4SL/Define CM Dict  xname=User.IO.Out.Brake_pedalFault  xmono=off  xtype=UInt  xdvaplace=None  xnstates=0  xfirststate=0  xinitial=0
  Define CM Dict55 : CarMaker4SL/Define CM Dict  xname=User.IO.Out.ESC_ABSValidity  xmono=off  xtype=UInt  xdvaplace=None  xnstates=0  xfirststate=0  xinitial=0
  Define CM Dict56 : CarMaker4SL/Define CM Dict  xname=User.IO.Out.ESC_ABSAlarmSig  xmono=off  xtype=UInt  xdvaplace=IO_Out  xnstates=0  xfirststate=0  xinitial=0
  Define CM Dict57 : CarMaker4SL/Define CM Dict  xname=User.IO.Out.ESC_FLWHeelPulVal  xmono=off  xtype=UInt  xdvaplace=None  xnstates=0  xfirststate=0  xinitial=0
  Define CM Dict58 : CarMaker4SL/Define CM Dict  xname=User.IO.Out.ESC_FRWHeelPulVal  xmono=off  xtype=UInt  xdvaplace=None  xnstates=0  xfirststate=0  xinitial=0
  Define CM Dict59 : CarMaker4SL/Define CM Dict  xname=User.IO.Out.ESC_RLWHeelPulVal  xmono=off  xtype=UInt  xdvaplace=None  xnstates=0  xfirststate=0  xinitial=0
  Define CM Dict6 : CarMaker4SL/Define CM Dict  xname=User.IO.Out.Mp5_TSR_Switch  xmono=off  xtype=UInt  xdvaplace=None  xnstates=0  xfirststate=0  xinitial=0
  Define CM Dict60 : CarMaker4SL/Define CM Dict  xname=User.IO.Out.ESC_RRWHeelSpdFlt  xmono=off  xtype=UInt  xdvaplace=None  xnstates=0  xfirststate=0  xinitial=0
  Define CM Dict61 : CarMaker4SL/Define CM Dict  xname=User.IO.Out.GW_TCU_ATFailure  xmono=off  xtype=Int  xdvaplace=None  xnstates=0  xfirststate=0  xinitial=0
  Define CM Dict62 : CarMaker4SL/Define CM Dict  xname=User.IO.Out.ESC_RRWHeelPulVal  xmono=off  xtype=UInt  xdvaplace=None  xnstates=0  xfirststate=0  xinitial=0
  Define CM Dict63 : CarMaker4SL/Define CM Dict  xname=User.IO.Out.ESC_FLWHeelSpdFlt  xmono=off  xtype=UInt  xdvaplace=None  xnstates=0  xfirststate=0  xinitial=0
  Define CM Dict64 : CarMaker4SL/Define CM Dict  xname=User.IO.Out.ESC_FRWHeelSpdFlt  xmono=off  xtype=UInt  xdvaplace=None  xnstates=0  xfirststate=0  xinitial=0
  Define CM Dict65 : CarMaker4SL/Define CM Dict  xname=User.IO.Out.ESC_RLWHeelSpdFlt  xmono=off  xtype=UInt  xdvaplace=None  xnstates=0  xfirststate=0  xinitial=0
  Define CM Dict66 : CarMaker4SL/Define CM Dict  xname=User.IO.Out.GW_TCU_SelATMode  xmono=off  xtype=UInt  xdvaplace=None  xnstates=0  xfirststate=0  xinitial=0
  Define CM Dict67 : CarMaker4SL/Define CM Dict  xname=User.IO.Out.GW_EMS_EngStatus  xmono=off  xtype=UInt  xdvaplace=None  xnstates=0  xfirststate=0  xinitial=0
  Define CM Dict68 : CarMaker4SL/Define CM Dict  xname=User.IO.Out.ESC_AEB_Status  xmono=off  xtype=UInt  xdvaplace=None  xnstates=0  xfirststate=0  xinitial=0
  Define CM Dict69 : CarMaker4SL/Define CM Dict  xname=User.IO.Out.ESC_AEB_Available  xmono=off  xtype=UInt  xdvaplace=None  xnstates=0  xfirststate=0  xinitial=0
  Define CM Dict7 : CarMaker4SL/Define CM Dict  xname=User.IO.Out.Mp5_ISA_Mode  xmono=off  xtype=UInt  xdvaplace=None  xnstates=0  xfirststate=0  xinitial=0
  Define CM Dict70 : CarMaker4SL/Define CM Dict  xname=User.IO.Out.ESC_ACC_Status  xmono=off  xtype=UInt  xdvaplace=None  xnstates=0  xfirststate=0  xinitial=0
  Define CM Dict71 : CarMaker4SL/Define CM Dict  xname=User.IO.Out.ESC_ACC_Available  xmono=off  xtype=UInt  xdvaplace=None  xnstates=0  xfirststate=0  xinitial=0
  Define CM Dict72 : CarMaker4SL/Define CM Dict  xname=User.IO.Out.BCM_FrontWiperSt  xmono=off  xtype=UInt  xdvaplace=None  xnstates=0  xfirststate=0  xinitial=0
  Define CM Dict73 : CarMaker4SL/Define CM Dict  xname=User.IO.Out.ACU_PassengerBelt  xmono=off  xtype=UInt  xdvaplace=None  xnstates=0  xfirststate=0  xinitial=0
  Define CM Dict74 : CarMaker4SL/Define CM Dict  xname=User.IO.Out.EMS_ACCctlAvail  xmono=off  xtype=UInt  xdvaplace=None  xnstates=0  xfirststate=0  xinitial=0
  Define CM Dict75 : CarMaker4SL/Define CM Dict  xname=User.IO.Out.EMS_ACC_Ihibited  xmono=off  xtype=UInt  xdvaplace=None  xnstates=0  xfirststate=0  xinitial=0
  Define CM Dict77 : CarMaker4SL/Define CM Dict  xname=User.IO.Out.EPB_EPBStatus  xmono=off  xtype=UInt  xdvaplace=None  xnstates=0  xfirststate=0  xinitial=0
  Define CM Dict78 : CarMaker4SL/Define CM Dict  xname=User.IO.Out.ACC_DesirHeadway  xmono=off  xtype=UInt  xdvaplace=None  xnstates=0  xfirststate=0  xinitial=0
  Define CM Dict79 : CarMaker4SL/Define CM Dict  xname=User.IO.Out.Fapa2Adas  xmono=off  xtype=Int  xdvaplace=None  xnstates=0  xfirststate=0  xinitial=0
  Define CM Dict8 : CarMaker4SL/Define CM Dict  xname=User.IO.Out.Mp5_LDWWarnMode  xmono=off  xtype=UInt  xdvaplace=None  xnstates=0  xfirststate=0  xinitial=0
  Define CM Dict81 : CarMaker4SL/Define CM Dict  xname=User.IO.Out.EPS_SteerHoldSt  xmono=off  xtype=UInt  xdvaplace=None  xnstates=0  xfirststate=0  xinitial=0
  Define CM Dict82 : CarMaker4SL/Define CM Dict  xname=User.IO.Out.BCM_BattVolt  xmono=off  xtype=UInt  xdvaplace=None  xnstates=0  xfirststate=0  xinitial=0
  Define CM Dict83 : CarMaker4SL/Define CM Dict  xname=User.IO.Out.Radar_State  xmono=off  xtype=UInt  xdvaplace=None  xnstates=0  xfirststate=0  xinitial=0
  Define CM Dict84 : CarMaker4SL/Define CM Dict  xname=User.IO.Out.ICAD_DecionState  xmono=off  xtype=UInt  xdvaplace=None  xnstates=0  xfirststate=0  xinitial=0
  Define CM Dict9 : CarMaker4SL/Define CM Dict  xname=User.IO.Out.MP5_ADAS_SegLmt  xmono=off  xtype=UInt  xdvaplace=None  xnstates=0  xfirststate=0  xinitial=0
  MP5_Cmd2Ctrl : Subsystem
  SensorStatus2Ctrl : Subsystem

== system MIL4L3_SW6_V1_20220211/CarMaker/IPG Vehicle/Brake/CreateBus Vhcl.Wheel.PT ==
  In : Inport
  BusCreator1 : BusCreator  Inputs=20
  Demux1 : Demux  Outputs=20
  Out : Outport
  wires:
  Demux1/20 -> BusCreator1/20  "Vhcl Trq_DriveSrc_trg d3"
  Demux1/19 -> BusCreator1/19  "Vhcl Trq_DriveSrc_trg d2"
  Demux1/18 -> BusCreator1/18  "Vhcl Trq_DriveSrc_trg d1"
  Demux1/17 -> BusCreator1/17  "Vhcl Trq_DriveSrc_trg d0"
  Demux1/16 -> BusCreator1/16  "Vhcl Wheel RR WhlBearing"
  Demux1/15 -> BusCreator1/15  "Vhcl Wheel RR Trq_T2W"
  Demux1/14 -> BusCreator1/14  "Vhcl Wheel RR Trq_BrakeReg_trg"
  Demux1/13 -> BusCreator1/13  "Vhcl Wheel RR Trq_Brake"
  Demux1/12 -> BusCreator1/12  "Vhcl Wheel RL WhlBearing"
  Demux1/11 -> BusCreator1/11  "Vhcl Wheel RL Trq_T2W"
  Demux1/10 -> BusCreator1/10  "Vhcl Wheel RL Trq_BrakeReg_trg"
  Demux1/9 -> BusCreator1/9  "Vhcl Wheel RL Trq_Brake"
  Demux1/8 -> BusCreator1/8  "Vhcl Wheel FR WhlBearing"
  Demux1/7 -> BusCreator1/7  "Vhcl Wheel FR Trq_T2W"
  Demux1/6 -> BusCreator1/6  "Vhcl Wheel FR Trq_BrakeReg_trg"
  Demux1/5 -> BusCreator1/5  "Vhcl Wheel FR Trq_Brake"
  Demux1/4 -> BusCreator1/4  "Vhcl Wheel FL WhlBearing"
  Demux1/3 -> BusCreator1/3  "Vhcl Wheel FL Trq_T2W"
  Demux1/2 -> BusCreator1/2  "Vhcl Wheel FL Trq_BrakeReg_trg"
  Demux1/1 -> BusCreator1/1  "Vhcl Wheel FL Trq_Brake"
  BusCreator1/1 -> Out/1
  In/1 -> Demux1/1

== system MIL4L3_SW6_V1_20220211/CarMaker/IPG Vehicle/CarAndTrailer/CarAndTrailerUpd ==
  Sync_In : Inport
  Vhcl.Steering : Inport  Port=2
  Vhcl.Motion : Inport  Port=3
  Vhcl.PoI : Inport  Port=4
  Vhcl.Wheel.FL : Inport  Port=5
  Vhcl.Wheel.FR : Inport  Port=6
  Vhcl.Wheel.RL : Inport  Port=7
  Vhcl.Wheel.RR : Inport  Port=8
  Car.Hitch.FrcTrq : Inport  Port=9
  Vhcl.Fr1A : Inport  Port=10
  CarAndTrailerUpd : S-Function  FunctionName=CM_Sfun  Parameters='CarAndTrUpd'  SFunctionDeploymentMode=off  EnableBusSupport=off
  CreateBus Brake.IF.In : Subsystem
  Sync_Out : Outport
  Brake.IF.In : Outport  Port=2
  wires:
  Vhcl.Fr1A/1 -> CarAndTrailerUpd/10  "user vehicle only"
  Vhcl.Steering/1 -> CarAndTrailerUpd/2
  Vhcl.Motion/1 -> CarAndTrailerUpd/3
  Vhcl.PoI/1 -> CarAndTrailerUpd/4
  Vhcl.Wheel.FL/1 -> CarAndTrailerUpd/5
  Vhcl.Wheel.FR/1 -> CarAndTrailerUpd/6
  Car.Hitch.FrcTrq/1 -> CarAndTrailerUpd/9
  Vhcl.Wheel.RR/1 -> CarAndTrailerUpd/8
  Vhcl.Wheel.RL/1 -> CarAndTrailerUpd/7
  CarAndTrailerUpd/2 -> CreateBus Brake.IF.In/1(In)
  CreateBus Brake.IF.In/1(Out) -> Brake.IF.In/1
  CarAndTrailerUpd/1 -> Sync_Out/1
  Sync_In/1 -> CarAndTrailerUpd/1

== system MIL4L3_SW6_V1_20220211/CarMaker/IPG Vehicle/CarAndTrailer/Forces ==
  Sync_In : Inport
  TireFL_In : Inport  Port=2
  TireFR_In : Inport  Port=3
  TireRL_In : Inport  Port=4
  TireRR_In : Inport  Port=5
  lSpring : Inport  Port=6
  vDamp : Inport  Port=7
  lStabi : Inport  Port=8
  lBuf : Inport  Port=9
  External Suspension Forces : Subsystem
  Tires : Subsystem
  Vehicle Forces : Subsystem
  Sync_Out : Outport
  Car.Virtual : Outport  Port=2
  Car.Aero : Outport  Port=3
  Car.Load : Outport  Port=4
  TireFL_Out : Outport  Port=5
  TireFR_Out : Outport  Port=6
  TireRL_Out : Outport  Port=7
  TireRR_Out : Outport  Port=8
  FSpring : Outport  Port=9
  FDamp : Outport  Port=10
  FStabi : Outport  Port=11
  FBuf : Outport  Port=12
  wires:
  lBuf/1 -> External Suspension Forces/5(lBuf)
  lStabi/1 -> External Suspension Forces/4(lStabi)
  vDamp/1 -> External Suspension Forces/3(vDamp)
  Tires/4(TireRR_Out) -> TireRR_Out/1
  Tires/3(TireRL_Out) -> TireRL_Out/1
  Tires/2(TireFR_Out) -> TireFR_Out/1
  Tires/1(TireFL_Out) -> TireFL_Out/1
  TireRR_In/1 -> Tires/5(TireRR_In)
  TireRL_In/1 -> Tires/4(TireRL_In)
  TireFR_In/1 -> Tires/3(TireFR_In)
  TireFL_In/1 -> Tires/2(TireFL_In)
  External Suspension Forces/4(FBuf) -> FBuf/1
  Sync_In/1 -> External Suspension Forces/1(Sync_In), Tires/1(Sync_In), Vehicle Forces/1(Sync_In)
  Vehicle Forces/1(Sync_Out) -> Sync_Out/1
  Vehicle Forces/2(Car.Virtual) -> Car.Virtual/1
  Vehicle Forces/3(Car.Aero) -> Car.Aero/1
  Vehicle Forces/4(Car.Load) -> Car.Load/1
  lSpring/1 -> External Suspension Forces/2(lSpring)
  External Suspension Forces/2(FDamp) -> FDamp/1
  External Suspension Forces/3(FStabi) -> FStabi/1
  External Suspension Forces/1(FSpring) -> FSpring/1

== system MIL4L3_SW6_V1_20220211/CarMaker/IPG Vehicle/CarAndTrailer/Kinematics ==
  Sync_In : Inport
  Steer.IF : Inport  Port=2
  Kinematics : S-Function  FunctionName=CM_Sfun  Parameters='Kinematics'  SFunctionDeploymentMode=off  EnableBusSupport=off
  Sync_Out : Outport
  TireFL_In : Outport  Port=2
  TireFR_In : Outport  Port=3
  TireRL_In : Outport  Port=4
  TireRR_In : Outport  Port=5
  lSpring : Outport  Port=6
  vDamp : Outport  Port=7
  lStabi : Outport  Port=8
  lBuf : Outport  Port=9
  wires:
  Kinematics/9 -> lBuf/1
  Kinematics/8 -> lStabi/1
  Kinematics/2 -> TireFL_In/1
  Kinematics/3 -> TireFR_In/1
  Kinematics/4 -> TireRL_In/1
  Kinematics/5 -> TireRR_In/1
  Kinematics/6 -> lSpring/1
  Kinematics/7 -> vDamp/1
  Sync_In/1 -> Kinematics/1
  Kinematics/1 -> Sync_Out/1
  Steer.IF/1 -> Kinematics/2

== system MIL4L3_SW6_V1_20220211/CarMaker/IPG Vehicle/CarAndTrailer/Kinetics ==
  Sync_In : Inport
  Car.Virtual : Inport  Port=2
  Car.Aero : Inport  Port=3
  Car.Load : Inport  Port=4
  TireFL.Out : Inport  Port=5
  TireFR.Out : Inport  Port=6
  TireRL.Out : Inport  Port=7
  TireRR.Out : Inport  Port=8
  FSpring : Inport  Port=9
  FDamp : Inport  Port=10
  FStabi : Inport  Port=11
  FBuf : Inport  Port=12
  Bus Creator : BusCreator  Inputs=4
  Bus Creator1 : BusCreator  Inputs=12
  Bus Creator2 : BusCreator  Inputs=6
  Bus Creator3 : BusCreator  Inputs=6
  Bus Creator4 : BusCreator  Inputs=4
  Demux : Demux  Outputs=12
  Demux1 : Demux  Outputs=6
  Demux2 : Demux  Outputs=6
  Demux3 : Demux
  Demux4 : Demux
  Kinetics : S-Function  FunctionName=CM_Sfun  Parameters='Kinetics'  SFunctionDeploymentMode=off  EnableBusSupport=off
  Sync_Out : Outport
  Trailer.Load : Outport  Port=2
  Car.Hitch : Outport  Port=3
  Car.Fr1 : Outport  Port=4
  Car.Trq_T2W : Outport  Port=5
  WheelCarrier.Misc : Outport  Port=6
  wires:
  FBuf/1 -> Kinetics/12
  Sync_In/1 -> Kinetics/1
  Kinetics/1 -> Sync_Out/1
  Car.Aero/1 -> Kinetics/3
  Car.Virtual/1 -> Kinetics/2
  Bus Creator1/1 -> Trailer.Load/1
  Demux/1 -> Bus Creator1/1  "Trailer Load_0 mass"
  Demux/2 -> Bus Creator1/2  "Trailer Load_0 tx"
  Demux/3 -> Bus Creator1/3  "Trailer Load_0 ty"
  Demux/4 -> Bus Creator1/4  "Trailer Load_0 tz"
  Kinetics/2 -> Demux/1
  Demux/5 -> Bus Creator1/5  "Trailer Load_1 mass"
  Demux/6 -> Bus Creator1/6  "Trailer Load_1 tx"
  Demux/7 -> Bus Creator1/7  "Trailer Load_1 ty"
  Demux/8 -> Bus Creator1/8  "Trailer Load_1 tz"
  Demux/9 -> Bus Creator1/9  "Trailer Load_2 mass"
  Demux/10 -> Bus Creator1/10  "Trailer Load_2 tx"
  Demux/11 -> Bus Creator1/11  "Trailer Load_2 ty"
  Demux/12 -> Bus Creator1/12  "Trailer Load_2 tz"
  Demux1/1 -> Bus Creator2/1  "Car Hitch tx"
  Demux1/2 -> Bus Creator2/2  "Car Hitch ty"
  Demux1/3 -> Bus Creator2/3  "Car Hitch tz"
  Demux1/4 -> Bus Creator2/4  "Car Hitch vx"
  Demux1/5 -> Bus Creator2/5  "Car Hitch vy"
  Demux1/6 -> Bus Creator2/6  "Car Hitch vz"
  Kinetics/3 -> Demux1/1
  Bus Creator2/1 -> Car.Hitch/1
  Demux2/1 -> Bus Creator3/1  "Car Fr1 rx"
  Demux2/2 -> Bus Creator3/2  "Car Fr1 ry"
  Demux2/3 -> Bus Creator3/3  "Car Fr1 rz"
  Demux2/4 -> Bus Creator3/4  "Car Fr1 rvx"
  Demux2/5 -> Bus Creator3/5  "Car Fr1 rvy"
  Demux2/6 -> Bus Creator3/6  "Car Fr1 rvz"
  Bus Creator3/1 -> Car.Fr1/1
  Kinetics/4 -> Demux2/1
  Car.Load/1 -> Kinetics/4
  Demux3/1 -> Bus Creator4/1  "car Susp FL GenInert2"
  Demux3/2 -> Bus Creator4/2  "car Susp FR GenInert2"
  Demux3/3 -> Bus Creator4/3  "car Susp FL GenFrc2"
  Demux3/4 -> Bus Creator4/4  "car Susp FR GenFrc2"
  Bus Creator4/1 -> WheelCarrier.Misc/1
  Bus Creator/1 -> Car.Trq_T2W/1
  Demux4/4 -> Bus Creator/4  "Car Trq_T2WRR"
  Demux4/3 -> Bus Creator/3  "Car Trq_T2WRL"
  Demux4/2 -> Bus Creator/2  "Car Trq_T2WFR"
  Demux4/1 -> Bus Creator/1  "Car Trq_T2WFL"
  TireFL.Out/1 -> Kinetics/5
  TireFR.Out/1 -> Kinetics/6
  TireRL.Out/1 -> Kinetics/7
  TireRR.Out/1 -> Kinetics/8
  FSpring/1 -> Kinetics/9
  FDamp/1 -> Kinetics/10
  FStabi/1 -> Kinetics/11
  Kinetics/6 -> Demux3/1
  Kinetics/5 -> Demux4/1

== system MIL4L3_SW6_V1_20220211/CarMaker/IPG Vehicle/CarAndTrailer/Steering ==
  note: When replacing the entire steering system,
      | be sure to add '-disablesteering' to the command line arguments
      | in the CarMaker Model Configuration block.
  Sync_In : Inport
  VhclCtrl.Steering : Inport  Port=2
  Bus Creator1 : BusCreator  Inputs=16
  Bus Creator2 : BusCreator  Inputs=5
  Demux : Demux  Outputs=21
  Steering : S-Function  FunctionName=CM_Sfun  Parameters='Steering'  SFunctionDeploymentMode=off  EnableBusSupport=off
  Terminator : Terminator
  Sync_Out : Outport
  Steer.IF : Outport  Port=2
  wires:
  Demux/21 -> Bus Creator2/5  "Steering IF R Inert"
  Demux/20 -> Bus Creator2/4  "Steering IF R Frc"
  Demux/19 -> Bus Creator2/3  "Steering IF L Inert"
  Demux/18 -> Bus Creator2/2  "Steering IF L Frc"
  Demux/17 -> Bus Creator2/1  "Steering IF SteerByTrq"
  Demux/16 -> Bus Creator1/16  "Steering IF R iSteer2q"
  Demux/15 -> Bus Creator1/15  "Steering IF R qpp"
  Demux/14 -> Bus Creator1/14  "Steering IF R qp"
  Demux/13 -> Bus Creator1/13  "Steering IF R q"
  Demux/12 -> Bus Creator1/12  "Steering IF L iSteer2q"
  Demux/11 -> Bus Creator1/11  "Steering IF L qpp"
  Demux/10 -> Bus Creator1/10  "Steering IF L qp"
  Demux/9 -> Bus Creator1/9  "Steering IF L q"
  Demux/8 -> Bus Creator1/8  "Steering IF AssistTrqPin"
  Demux/7 -> Bus Creator1/7  "Steering IF AssistTrqCol"
  Demux/6 -> Bus Creator1/6  "Steering IF AssistFrc"
  Demux/5 -> Bus Creator1/5  "Steering IF TrqStatic"
  Demux/4 -> Bus Creator1/4  "Steering IF Trq"
  Demux/3 -> Bus Creator1/3  "Steering IF AngAcc"
  Demux/2 -> Bus Creator1/2  "Steering IF AngVel"
  Demux/1 -> Bus Creator1/1  "Steering IF Ang"
  Bus Creator1/1 -> Steer.IF/1
  Steering/2 -> Demux/1
  Bus Creator2/1 -> Terminator/1  "Steer IF (in)"
  VhclCtrl.Steering/1 -> Steering/2
  Steering/1 -> Sync_Out/1
  Sync_In/1 -> Steering/1

== system MIL4L3_SW6_V1_20220211/CarMaker/IPG Vehicle/CarAndTrailer/Trailer ==
  Sync_In : Inport
  Trailer.Load : Inport  Port=2
  Car.Hitch : Inport  Port=3
  Car.Fr1 : Inport  Port=4
  Car.Trq_T2W : Inport  Port=5
  WheelCarrier.Misc : Inport  Port=6
  CreateBus Car.Hitch.FrcTrq : Subsystem
  CreateBus Vhcl.Motion : Subsystem
  CreateBus Vhcl.PoI : Subsystem
  CreateBus Vhcl.Steering : Subsystem
  CreateBus Vhcl.Wheel.FL : Subsystem
  CreateBus Vhcl.Wheel.FR : Subsystem
  CreateBus Vhcl.Wheel.RL : Subsystem
  CreateBus Vhcl.Wheel.RR : Subsystem
  Trailer : S-Function  FunctionName=CM_Sfun  Parameters='Trailer'  SFunctionDeploymentMode=off  EnableBusSupport=off
  Sync_Out : Outport
  Vhcl.Steering : Outport  Port=2
  Vhcl.Motion : Outport  Port=3
  Vhcl.PoI : Outport  Port=4
  Vhcl.Wheel.FL : Outport  Port=5
  Vhcl.Wheel.FR : Outport  Port=6
  Vhcl.Wheel.RL : Outport  Port=7
  Vhcl.Wheel.RR : Outport  Port=8
  Car.Hitch.FrcTrq : Outport  Port=9
  wires:
  Trailer/2 -> CreateBus Vhcl.Steering/1(In1)
  CreateBus Vhcl.Steering/1(Out1) -> Vhcl.Steering/1  "Vhcl.Steering"
  Trailer/3 -> CreateBus Vhcl.Motion/1(In1)
  Trailer/4 -> CreateBus Vhcl.PoI/1(In1)
  Trailer/5 -> CreateBus Vhcl.Wheel.FL/1(In1)
  Trailer/6 -> CreateBus Vhcl.Wheel.FR/1(In1)
  Trailer/7 -> CreateBus Vhcl.Wheel.RL/1(In1)
  Trailer/9 -> CreateBus Car.Hitch.FrcTrq/1(In1)
  Trailer/8 -> CreateBus Vhcl.Wheel.RR/1(In1)
  CreateBus Vhcl.Wheel.RR/1(Out1) -> Vhcl.Wheel.RR/1  "Vhcl.Wheel.RR"
  CreateBus Vhcl.Wheel.RL/1(Out1) -> Vhcl.Wheel.RL/1  "Vhcl.Wheel.RL"
  CreateBus Vhcl.Wheel.FR/1(Out1) -> Vhcl.Wheel.FR/1  "Vhcl.Wheel.FR"
  CreateBus Vhcl.Wheel.FL/1(Out1) -> Vhcl.Wheel.FL/1  "Vhcl.Wheel.FL"
  CreateBus Vhcl.PoI/1(Out1) -> Vhcl.PoI/1  "Vhcl.PoI"
  CreateBus Vhcl.Motion/1(Out1) -> Vhcl.Motion/1  "Vhcl.Motion"
  Car.Trq_T2W/1 -> Trailer/5
  WheelCarrier.Misc/1 -> Trailer/6
  CreateBus Car.Hitch.FrcTrq/1(Out1) -> Car.Hitch.FrcTrq/1  "Car.Hitch.FrcTrq"
  Car.Fr1/1 -> Trailer/4
  Car.Hitch/1 -> Trailer/3
  Trailer.Load/1 -> Trailer/2
  Trailer/1 -> Sync_Out/1
  Sync_In/1 -> Trailer/1
